simulink model "stereo_ibvs_core_before_04_kinematics_20260723_210007"  (R2025b)
settings: Solver=FixedStepDiscrete  StartTime=0.0  StopTime=inf  FixedStep=cfg.Ts  RelTol=1e-3
InitFcn:
  | cfgValid__=evalin('base','exist(''cfg'',''var'')==1 && isstruct(cfg) && all(isfield(cfg,{''Ts'',''robot'',''qInitial'',''zoomInitialSteps'',''cameraIntrinsicsStage1'',''rhoD'',''stereoBaseline'',''centerDesired'',''Kc'',''lambdaC'',''qMin'',''qMax'',''qLimitSoftMargin'',''qDotAlgorithmMax'',''stage1CalibrationReady''}))');if ~cfgValid__,modelFile__=get_param(bdroot,'FileName');modelDir__=fileparts(modelFile__);config1__=fullfile(modelDir__,'stereo_ibvs_config.m');config2__=fullfile(fileparts(modelDir__),'config','stereo_ibvs_config.m');if isfile(config1__),run(config1__);elseif isfile(config2__),run(config2__);else,error('StereoIBVS:ConfigNotFound','找不到stereo_ibvs_config.m。');end;end;clear cfgValid__ modelFile__ modelDir__ config1__ config2__
undefined symbols (not defined in the file): cfg
(part 2 of 2)

== matlab function stereo_ibvs_core_before_04_kinematics_20260723_210007/07_Arm_Priority_Controller/Final Arm Priority Controller ==
  data: q input double size=[7 1]; qDotCmd output double size=[7 1]; cLMeasured input double size=[2 1]; rhoHatL input double size=[1 1]; vHatLeft input double size=[3 1]; JL input double size=[6 7]; cLd input double size=[2 1]; rhoD input double size=[1 1]; validLeft input double size=[1 1]; ekfPredictionValid input double size=[1 1]; centerEnable input double size=[1 1]; depthEnable input double size=[1 1]; armEnable input double size=[1 1]; depthTaskWeight input double size=[1 1]; cfg_numericalEpsilon input double size=[1 1]; cfg_robustEnable input double size=[1 1]; cfg_betaC input double size=[1 1]; cfg_epsilonC input double size=[1 1]; cfg_Kc input double size=[2 2]; cfg_lambdaC input double size=[1 1]; cfg_betaRho input double size=[1 1]; cfg_epsilonRho input double size=[1 1]; cfg_kRho input double size=[1 1]; cfg_lambdaRho input double size=[1 1]; cfg_nullspaceEnable input double size=[1 1]; cfg_kNull input double size=[1 1]; cfg_qMid input double size=[7 1]; cfg_leftOnlyCenterControlEnable input double size=[1 1]; centerError output double size=[2 1]; depthError output double size=[1 1]; rcondJc output double size=[1 1]; rcondArho output double size=[1 1]; qDotCenter output double size=[7 1]; qDotDepthRaw output double size=[7 1]; qDotDepthWeighted output double size=[7 1]; qDotNullUsed output double size=[7 1]
function [qDotCmd,centerError,depthError,rcondJc,rcondArho,qDotCenter,qDotDepthRaw,qDotDepthWeighted,qDotNullUsed] = ...
    fcn(q,cLMeasured,rhoHatL,vHatLeft,JL,cLd,rhoD,validLeft,ekfPredictionValid,centerEnable,depthEnable,armEnable,depthTaskWeight, ...
    cfg_numericalEpsilon,cfg_robustEnable,cfg_betaC,cfg_epsilonC,cfg_Kc,cfg_lambdaC,cfg_betaRho,cfg_epsilonRho,cfg_kRho,cfg_lambdaRho,cfg_nullspaceEnable,cfg_kNull,cfg_qMid,cfg_leftOnlyCenterControlEnable)
%#codegen
% 代码作用：
% 左相机归一化中心为主任务，逆深度为次任务。
% 支持目标速度前馈、鲁棒项、阻尼伪逆和关节中位零空间任务。

qDotCmd = zeros(7,1);
centerError = zeros(2,1);
depthError = 0;
rcondJc = 0;
rcondArho = 0;
qDotCenter = zeros(7,1);
qDotDepthRaw = zeros(7,1);
qDotDepthWeighted = zeros(7,1);
qDotNullUsed = zeros(7,1);

x = cLMeasured(1);
y = cLMeasured(2);
rho = rhoD;
vFeed = zeros(3,1);

if ekfPredictionValid > 0.5 && ...
        isfinite(rhoHatL) && rhoHatL > 0 && ...
        all(isfinite(vHatLeft))
    rho = max(rhoHatL,cfg_numericalEpsilon);
    vFeed = vHatLeft;
end

centerError = [x;y] - cLd;
depthError = rho - rhoD;

Lc = [
    -rho, 0, x*rho, x*y, -(1+x*x), y
    0, -rho, y*rho, 1+y*y, -x*y, -x
];

Hc = rho*[1 0 -x;0 1 -y];
bhatC = Hc*vFeed;
Jc = Lc*JL;

rc = zeros(2,1);
if cfg_robustEnable > 0.5
    rc = cfg_betaC*centerError / ...
        (sqrt(centerError'*centerError)+cfg_epsilonC);
end

nuC = -cfg_Kc*centerError - bhatC - rc;
Gc = Jc*Jc' + cfg_lambdaC^2*eye(2);
JcSharp = Jc'/Gc;
qC = JcSharp*nuC;
Nc = eye(7)-JcSharp*Jc;
rcondJc = det(Gc) / ...
    (trace(Gc)*trace(Gc)+cfg_numericalEpsilon);
qDotCenter = qC;

Lrho = [0 0 rho*rho rho*y -rho*x 0];
Hrho = [0 0 -rho*rho];
Jrho = Lrho*JL;
bhatRho = Hrho*vFeed;

rr = 0;
if cfg_robustEnable > 0.5
    rr = cfg_betaRho*depthError / ...
        (abs(depthError)+cfg_epsilonRho);
end

nuRho = -cfg_kRho*depthError-bhatRho-rr;
A = Jrho*Nc;
denom = A*A'+cfg_lambdaRho^2;
rcondArho = denom/(1+denom);

w = min(max(depthTaskWeight,0),1) * ...
    double(ekfPredictionValid > 0.5);
qDotDepthRaw = Nc*A'*((nuRho-Jrho*qC)/denom);
qDotDepthWeighted = w*qDotDepthRaw;

qDot0 = zeros(7,1);
if cfg_nullspaceEnable > 0.5
    qDot0 = -cfg_kNull*(q-cfg_qMid);
end

ArhoDagger = A'/denom;
NcRho = Nc*(eye(7)-ArhoDagger*A);
Nnull = (1-w)*Nc+w*NcRho;
qDotNullUsed = Nnull*qDot0;

if centerEnable > 0.5
    qDotCmd = qDotCenter+qDotNullUsed;
end

if centerEnable > 0.5 && depthEnable > 0.5
    qDotCmd = qDotCenter+qDotDepthWeighted+qDotNullUsed;
end

if centerEnable <= 0.5 && depthEnable > 0.5
    d = Jrho*Jrho'+cfg_lambdaRho^2;
    qDotDepthRaw = Jrho'*(nuRho/d);
    qDotDepthWeighted = w*qDotDepthRaw;
    qDotCenter = zeros(7,1);
    qDotNullUsed = zeros(7,1);
    qDotCmd = qDotDepthWeighted;
end

centerAllowed = validLeft > 0.5 && ...
    cfg_leftOnlyCenterControlEnable > 0.5;

if ~centerAllowed || armEnable <= 0.5
    qDotCmd = zeros(7,1);
    qDotCenter = zeros(7,1);
    qDotDepthWeighted = zeros(7,1);
    qDotNullUsed = zeros(7,1);
end

if any(~isfinite(qDotCmd))
    qDotCmd = zeros(7,1);
end
end
